simulink model "CRUISE_CONTROL_APPLICATION"  (R2021b)
settings: Solver=FixedStepAuto  StartTime=0.0  StopTime=25  RelTol=1e-3
PreLoadFcn:
  | clearvars;
  | m=1000;
  | b=50;
  | u=100;
  | Ts=0.01;
  | kp=800;
  | ki=40;
  | kd=0;
  | up=7000;
settings Model: Creator=sudhir  LastModifiedBy=sudhir

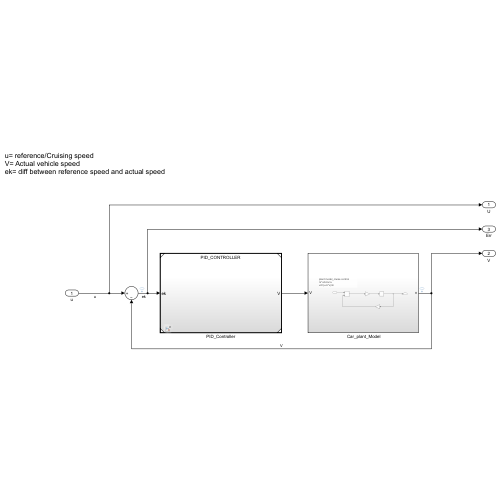
[thumbnail: Simulink's stored preview of the top-level diagram]
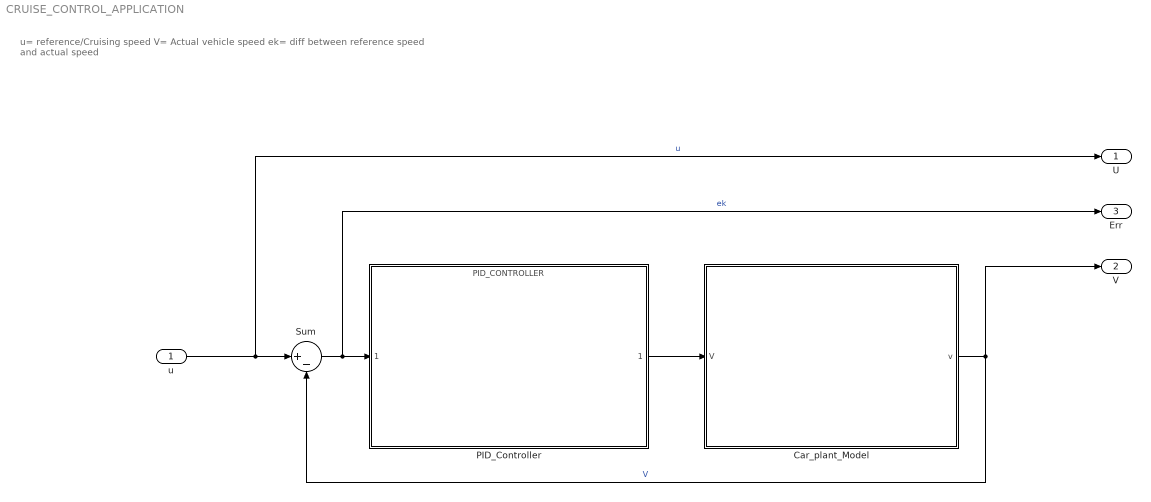
== system CRUISE_CONTROL_APPLICATION ==
  note: u= reference/Cruising speed
      | V= Actual vehicle speed
      | ek= diff between reference speed and actual speed
  u : Inport
  " Car_plant_Model" : Subsystem
  PID_Controller : ModelReference  ModelNameDialog=PID_CONTROLLER.slx  SimulationMode=Normal  ModelReferenceVersion=1.43
  Sum : Sum  Inputs=|+-
  U : Outport
  V : Outport  Port=2
  Err : Outport  Port=3
  wires:
  PID_Controller/1 -> " Car_plant_Model"/1(V)
  u/1 -> U/1, Sum/1  "u"
  Sum/1 -> Err/1, PID_Controller/1  "ek"
  " Car_plant_Model"/1(v) -> V/1, Sum/2  "V"

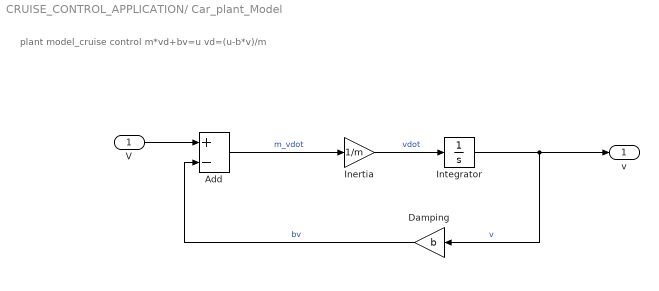
== system CRUISE_CONTROL_APPLICATION/ Car_plant_Model ==
  note: plant model_cruise control
      | m*vd+bv=u
      | vd=(u-b*v)/m
  V : Inport
  Add : Sum  Inputs=+-
  Damping : Gain  Gain=b
  Inertia : Gain  Gain=1/m
  Integrator : Integrator
  v : Outport
  wires:
  Inertia/1 -> Integrator/1  "vdot"
  Integrator/1 -> v/1, Damping/1  "v"
  Damping/1 -> Add/2  "bv"
  Add/1 -> Inertia/1  "m_vdot"
  V/1 -> Add/1
